simulink model "aeroSurface_th"  (R2018b)
settings: Solver=VariableStepAuto  StartTime=0.0  StopTime=0  RelTol=1e-3
values from neighbouring files (symbols this model uses):
  defAng = 1*pi/180    (= 0.0174532925199)    [aeroSurface_ts1.m]    (also in aeroSurface_ts2.m = 0)
  dynPress = 1    [aeroSurface_ts1.m]    (also in aeroSurface_ts2.m)
  uAppBody = uAppBody/sqrt(sum(uAppBody.^2))    [aeroSurface_ts1.m]    (also in aeroSurface_ts2.m)
libraries: aeroSurface_ul x2
settings Model: Creator=mcobb  LastModifiedBy=mcobb

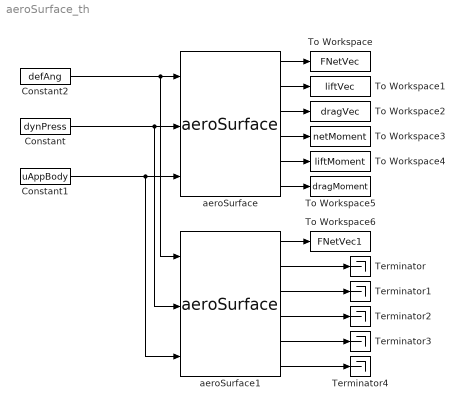
== system aeroSurface_th ==
  Constant : Constant  Value=dynPress
  Constant1 : Constant  Value=uAppBody
  Constant2 : Constant  Value=defAng
  Terminator{,1..4} (5 alike) : Terminator
  To Workspace : ToWorkspace  VariableName=FNetVec  SaveFormat=Timeseries  SampleTime=-1
  To Workspace1 : ToWorkspace  VariableName=liftVec  SaveFormat=Timeseries  SampleTime=-1
  To Workspace2 : ToWorkspace  VariableName=dragVec  SaveFormat=Timeseries  SampleTime=-1
  To Workspace3 : ToWorkspace  VariableName=netMoment  SaveFormat=Timeseries  SampleTime=-1
  To Workspace4 : ToWorkspace  VariableName=liftMoment  SaveFormat=Timeseries  SampleTime=-1
  To Workspace5 : ToWorkspace  VariableName=dragMoment  SaveFormat=Timeseries  SampleTime=-1
  To Workspace6 : ToWorkspace  VariableName=FNetVec1  SaveFormat=Timeseries  SampleTime=-1
  aeroSurface : aeroSurface_ul/aeroSurface  rAeroCent=aeroCenterVec  uSpan=spanRotationVec  uChord=chordDirectionVec  airfoilSelection=NACA-0009 9.0% smoothed_T1_Re1.000_M0.00_N9.0.txt  ARef=refArea  AR=8  OE=0.8  useFit=on  clFitLims=[-10 10]  clFitOrder=1  cdFitLims=[-10 10]  cdFitOrder=2
      link override LiftCoefficients: BreakpointsForDimension1=aeroTable.alpha  Table=aeroTable.cl
  aeroSurface1 : aeroSurface_ul/aeroSurface  rAeroCent=aeroCenterVec  uSpan=spanRotationVec  uChord=chordDirectionVec  airfoilSelection=NACA 4412_T1_Re5.085_M0.00_N9.0.txt  ARef=refArea  AR=8  OE=0.8  useFit=off  clFitLims=[-10 10]  clFitOrder=1  cdFitLims=[-10 10]  cdFitOrder=2
      link override LiftCoefficients: BreakpointsForDimension1=aeroTable.alpha  Table=aeroTable.cl
  wires:
  Constant/1 -> aeroSurface1/2, aeroSurface/2
  Constant1/1 -> aeroSurface1/3, aeroSurface/3
  aeroSurface/1 -> To Workspace/1
  aeroSurface/6 -> To Workspace5/1
  aeroSurface/5 -> To Workspace4/1
  aeroSurface/4 -> To Workspace3/1
  aeroSurface/3 -> To Workspace2/1
  aeroSurface/2 -> To Workspace1/1
  Constant2/1 -> aeroSurface/1, aeroSurface1/1
  aeroSurface1/1 -> To Workspace6/1
  aeroSurface1/2 -> Terminator/1
  aeroSurface1/3 -> Terminator1/1
  aeroSurface1/4 -> Terminator2/1
  aeroSurface1/5 -> Terminator3/1
  aeroSurface1/6 -> Terminator4/1
